simulink model "ex3_sim1"  (R2018b)
settings: Solver=ode45  StartTime=0.0  StopTime=2  MaxStep=0.01  RelTol=1e-3
undefined symbols (not defined in the file): Ad, Ar, denC, denH, denP, denQ, numC, numH, numP, numQ, t0d, t0r, Ts
settings Model: Creator=riccardo  LastModifiedBy=riccardo

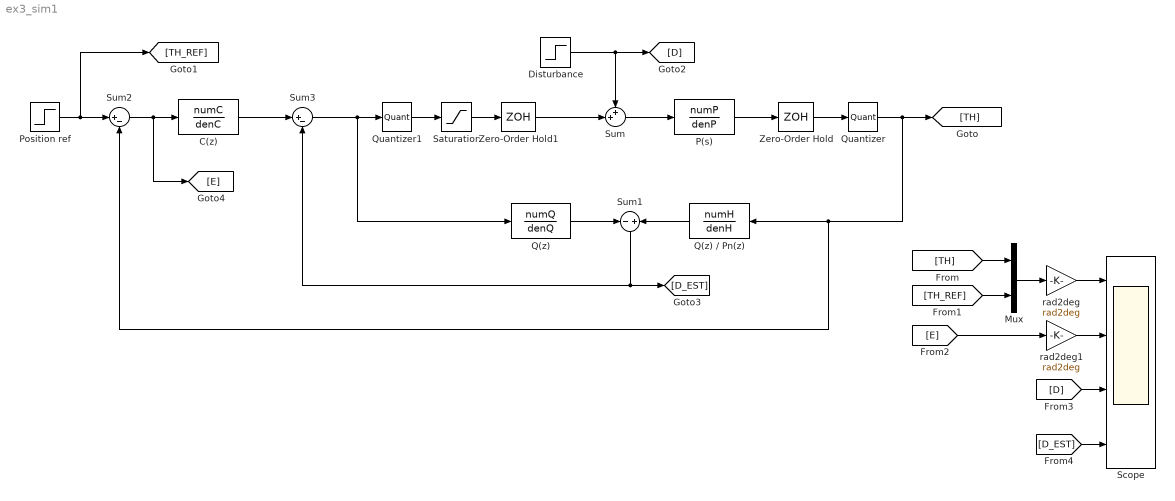
== system ex3_sim1 ==
  C(z) : DiscreteTransferFcn  Numerator=numC  Denominator=denC  SampleTime=Ts
  Disturbance : Step  Time=t0d  After=Ad  SampleTime=0
  Mux : Mux  Inputs=2
  P(s) : TransferFcn  Numerator=numP  Denominator=denP
  Position ref : Step  Time=t0r  After=Ar  SampleTime=Ts
  Q(z) : DiscreteTransferFcn  Numerator=numQ  Denominator=denQ  SampleTime=Ts
  Q(z) / Pn(z) : DiscreteTransferFcn  Numerator=numH  Denominator=denH  SampleTime=Ts
  Quantizer : Quantizer  QuantizationInterval=2*pi/2000
  Quantizer1 : Quantizer  QuantizationInterval=20/2^10
  Saturation : Saturate  UpperLimit=10  LowerLimit=-10
  Scope : Scope  NumInputPorts=4
  Sum : Sum  Inputs=++|
  Sum1 : Sum  Inputs=-+
  Sum2 : Sum  Inputs=|+-
  Sum3 : Sum  Inputs=|+-
  Zero-Order Hold : ZeroOrderHold  SampleTime=Ts
  Zero-Order Hold1 : ZeroOrderHold  SampleTime=Ts
  rad2deg : Gain  Gain=rad2deg
  rad2deg1 : Gain  Gain=rad2deg
  wires:
  Sum/1 -> P(s)/1
  P(s)/1 -> Zero-Order Hold/1
  Q(z)/1 -> Sum1/1
  Q(z) / Pn(z)/1 -> Sum1/2
  Saturation/1 -> Zero-Order Hold1/1
  Sum2/1 -> [E], C(z)/1
  Position ref/1 -> [TH_REF], Sum2/1
  Sum3/1 -> Q(z)/1, Quantizer1/1
  Mux/1 -> rad2deg/1
  [TH] -> Mux/1
  [TH_REF] -> Mux/2
  [E] -> rad2deg1/1
  rad2deg/1 -> Scope/1
  Sum1/1 -> Sum3/2, [D_EST]
  C(z)/1 -> Sum3/1
  Disturbance/1 -> [D], Sum/1
  Zero-Order Hold/1 -> Quantizer/1
  Quantizer/1 -> Q(z) / Pn(z)/1, Sum2/2, [TH]
  Zero-Order Hold1/1 -> Sum/2
  Quantizer1/1 -> Saturation/1
  rad2deg1/1 -> Scope/2
  [D] -> Scope/3
  [D_EST] -> Scope/4
